simulink model "mcb_pmsm_foc_I2C_f28379d"  (R2023b)
settings: Solver=FixedStepDiscrete  StartTime=0.0  StopTime=4  RelTol=1e-3  EnableMultiTasking=on
InitFcn:
  | mcb_pmsm_foc_I2C_f28379d_data;
values from neighbouring files (symbols this model uses):
  dataType = 'single'    [mcb_pmsm_foc_I2C_f28379d_data.m]
  inverter = mcb_updateInverterParameters(pmsm,inverter,target)    [mcb_pmsm_foc_I2C_f28379d_data.m]
  PI_params = mcb_SetControllerParameters(pmsm,inverter,PU_System,T_pwm,Ts,Ts_speed)    [mcb_pmsm_foc_I2C_f28379d_data.m]
  pmsm = mcb_SetPMSMMotorParameters("SF2804")    [mcb_pmsm_foc_I2C_f28379d_data.m]
  PU_System = mcb_SetPUSystem(pmsm,inverter)    [mcb_pmsm_foc_I2C_f28379d_data.m]
  target = mcb_SetProcessorDetails('F28379D',PWM_frequency)    [mcb_pmsm_foc_I2C_f28379d_data.m]
  Ts = T_pwm    (= 5e-05)    [mcb_pmsm_foc_I2C_f28379d_data.m]
  Ts_motor = T_pwm/2    (= 2.5e-05)    [mcb_pmsm_foc_I2C_f28379d_data.m]
  Ts_sensor = 20*Ts    (= 0.001)    [mcb_pmsm_foc_I2C_f28379d_data.m]
  Ts_simulink = T_pwm/2    (= 2.5e-05)    [mcb_pmsm_foc_I2C_f28379d_data.m]
  Ts_speed = 10*Ts    (= 0.0005)    [mcb_pmsm_foc_I2C_f28379d_data.m]
undefined symbols (not defined in the file or in its folder): acceleration, DiscIntNeverNeededParam, Down, GPTRIP1SEL, GPTRIP2SEL, Speed_openLoop_PU, TZ1, TZ2, Up
libraries: c280xlib x14, simulink x12, mcbcontrolslib x9, c2802xlib x7, slpidlib x5, c2837xDlib x4, mcbpositiondecoderlib x3, canmsglib x2, svdschedulerlib x2, dspsigops x1, svdutilitieslib x1, mcbplantlib x1
(part 1 of 3)
settings Model: ExtModeTrigDuration=8  Creator=The MathWorks, Inc.  LastModifiedBy=13571
settings SolverCC: AlgebraicLoopSolver=TrustRegion  AutoInsertRateTranBlk=on  MaxZcPerStep=1
settings OptimizationCC: DefaultParameterBehavior=Inlined  DefaultUnderspecifiedDataType=single  OptimizeBlockIOStorage=off  ReuseModelBlockBuffer=off  EnhancedBackFolding=on  InitFltsAndDblsToZero=on  NoFixptDivByZeroProtection=on  EfficientFloat2IntCast=on  EfficientMapNaN2IntZero=off  MaxStackSize=1024  OptimizeBlockOrder=speed  DifferentSizesBufferReuse=on  DenormalBehavior=FlushToZero  EfficientTunableParamExpr=on
settings DebuggingCC: MultiTaskDSMMsg=none  ParameterPrecisionLossMsg=none  ParameterTunabilityLossMsg=error  UnconnectedInputMsg=warning  UnconnectedOutputMsg=warning  UnconnectedLineMsg=warning
settings HardwareCC: ProdBitPerChar=16  ProdBitPerInt=16  ProdBitPerPointer=32  ProdBitPerSizeT=32  ProdBitPerPtrDiffT=32  ProdLargestAtomicInteger=Integer  ProdLargestAtomicFloat=None  ProdWordSize=16  ProdLongLongMode=on  ProdHWDeviceType=Texas Instruments->C2000
settings ModelReferenceCC: EnableRefExpFcnMdlSchedulingChecks=on
settings SFSimCC: MATLABDynamicMemAlloc=off
settings RTWCC: Description=Embedded Coder  SystemTargetFile=ert.tlc  HardwareBoard=TI Delfino F28379D LaunchPad  TemplateMakefile=ert_default_tmf  GenerateReport=on  Toolchain=Texas Instruments Code Composer Studio (C2000)  DLArmComputeVersion=19.05
settings CodeAppCC: IgnoreCustomStorageClasses=off  StateflowObjectComments=on
settings ERTTargetCC: CodeReplacementLibrary=TI C28x  ExtModeStaticAllocSize=10000  ConvertIfToSwitch=off  SuppressUnreachableDefaultCases=off  MemSecPackage=tic2000demospkg

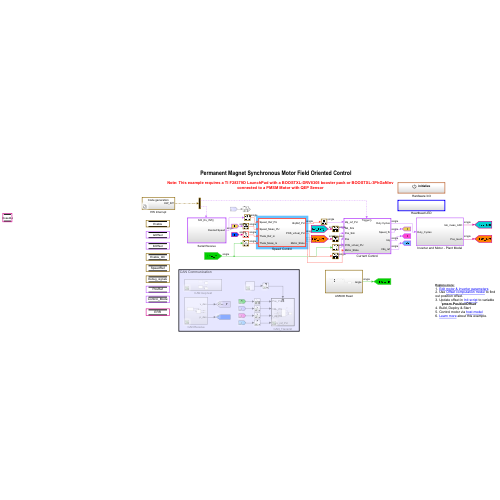
[thumbnail: Simulink's stored preview of the top-level diagram]
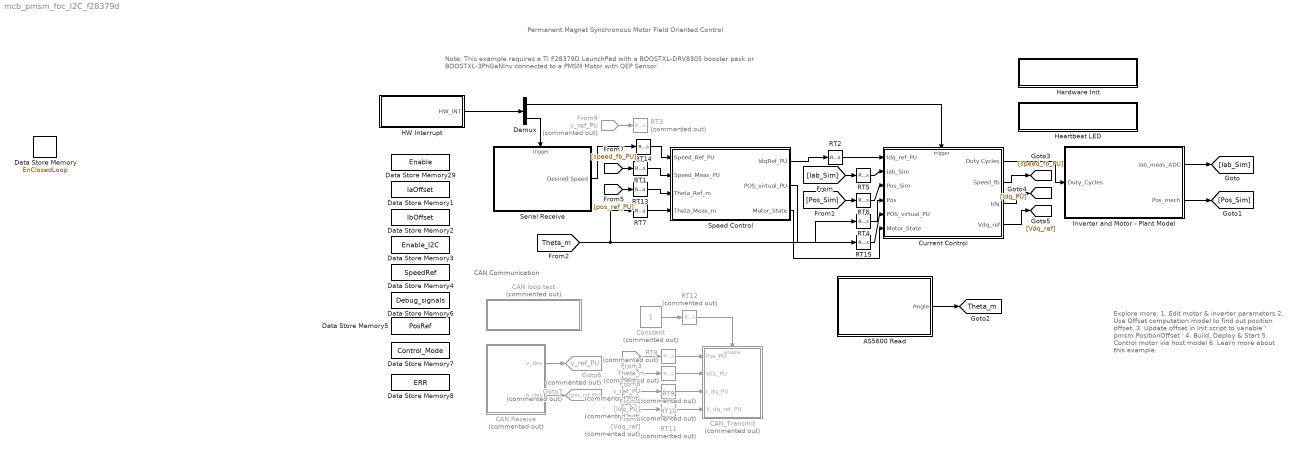
== system mcb_pmsm_foc_I2C_f28379d ==
  note: CAN Communication
  note: Note: This example requires a TI F28379D LaunchPad with a BOOSTXL-DRV8305 booster pack or BOOSTXL-3PhGaNInv
      | connected to a PMSM Motor with QEP Sensor
  note: Permanent Magnet Synchronous Motor Field Oriented Control
  note: Explore more:
      | 1. Edit motor & inverter parameters
      | 2. Use Offset computation model to find out position offset.
      | 3. Update offset in Init script to variable ' pmsm.PositionOffset '
      | 4. Build, Deploy & Start
      | 5. Control motor via host model
      | 6. Learn more about this example.
  AS5600 Read : Subsystem
  CAN Receive : Subsystem  Commented=on
  CAN loop test : Subsystem  Commented=on
  CAN_Transmit : Subsystem  Commented=on
  Constant : Constant  Commented=on  SampleTime=15e-2
  Current Control : Subsystem
      settings: RTWSystemCode=Nonreusable function
  Data Store Memory1 : DataStoreMemory  DataStoreName=IaOffset  ReadBeforeWriteMsg=warning  WriteAfterWriteMsg=warning  WriteAfterReadMsg=warning  InitialValue=inverter.CtSensAOffset  ShowAdditionalParam=off
  Data Store Memory2 : DataStoreMemory  DataStoreName=IbOffset  ReadBeforeWriteMsg=warning  WriteAfterWriteMsg=warning  WriteAfterReadMsg=warning  InitialValue=inverter.CtSensBOffset  ShowAdditionalParam=off
  Data Store Memory29 : DataStoreMemory  DataStoreName=Enable  ReadBeforeWriteMsg=warning  WriteAfterWriteMsg=warning  WriteAfterReadMsg=warning  ShowAdditionalParam=off  OutDataTypeStr=boolean
  Data Store Memory3 : DataStoreMemory  DataStoreName=Enable_I2C  ReadBeforeWriteMsg=warning  WriteAfterWriteMsg=warning  WriteAfterReadMsg=warning  ShowAdditionalParam=off  OutDataTypeStr=boolean
  Data Store Memory4 : DataStoreMemory  DataStoreName=SpeedRef  ShowAdditionalParam=off
  Data Store Memory5 : DataStoreMemory  DataStoreName=PosRef  ShowAdditionalParam=off
  Data Store Memory6 : DataStoreMemory  DataStoreName=Debug_signals  ReadBeforeWriteMsg=warning  WriteAfterWriteMsg=warning  WriteAfterReadMsg=warning  InitialValue=5  ShowAdditionalParam=off  OutDataTypeStr=uint16
  Data Store Memory7 : DataStoreMemory  DataStoreName=Control_Mode  ShowAdditionalParam=off
  Data Store Memory8 : DataStoreMemory  DataStoreName=ERR  ShowAdditionalParam=off
  Data Store Memory : DataStoreMemory  DataStoreName=EnClosedLoop  WriteAfterWriteMsg=warning  ShowAdditionalParam=off
  Demux : Demux  Outputs=2
  From3 : From  Commented=on  GotoTag=Theta_m  TagVisibility=global
  From4 : From  Commented=on  GotoTag=Idq_PU
  From6 : From  Commented=on  GotoTag=Vdq_ref
  From8 : From  Commented=on  GotoTag=v_ref_PU  TagVisibility=global
  From9 : From  Commented=on  GotoTag=v_ref_PU  TagVisibility=global
  Goto6 : Goto  Commented=on  GotoTag=v_ref_PU  TagVisibility=global
  Goto7 : Goto  Commented=on  GotoTag=pos_ref_PU
  HW Interrupt : Subsystem  Variant=on  VariantControlMode=sim codegen switching
  Hardware Init : Subsystem  TreatAsAtomicUnit=on
  Heartbeat LED : Subsystem  TreatAsAtomicUnit=on
  Inverter and Motor - Plant Model : Subsystem
  RT1 : RateTransition  Deterministic=off  OutPortSampleTime=Ts_speed
  RT{8..11} (4 alike) : RateTransition  Commented=on  Deterministic=off
  RT12 : RateTransition  Commented=on  Deterministic=off  OutPortSampleTime=1e-1
  RT13 : RateTransition  Deterministic=off  OutPortSampleTime=Ts_speed
  RT14 : RateTransition  Deterministic=off  OutPortSampleTime=Ts_speed
  RT{2,4..7,15} (6 alike) : RateTransition  Deterministic=off
  RT3 : RateTransition  Commented=on  Deterministic=off  OutPortSampleTime=Ts_speed
  Serial Receive : Subsystem  SystemSampleTime=1e-3
  Speed Control : Subsystem  TreatAsAtomicUnit=on  SystemSampleTime=Ts_speed
  tag scope: Theta_m=global
  wires:
  HW Interrupt/1(HW_INT) -> Demux/1
  RT2/1 -> Current Control/1(Idq_ref_PU)
  Demux/1 -> Current Control/Trigger
  Current Control/1(Duty Cycles) -> Inverter and Motor - Plant Model/1(Duty_Cycles)
  Demux/2 -> Serial Receive/Trigger
  Speed Control/1(IdqRef_PU) -> RT2/1
  RT1/1 -> Speed Control/2(Speed_Meas_PU)
  Inverter and Motor - Plant Model/2(Pos_mech) -> [Pos_Sim]
  Inverter and Motor - Plant Model/1(Iab_meas_ADC) -> [Iab_Sim]
  RT6/1 -> Current Control/3(Pos_Sim)
  [Iab_Sim] -> RT5/1
  RT5/1 -> Current Control/2(Iab_Sim)
  [Pos_Sim] -> RT6/1
  AS5600 Read/1(Angle) -> [Theta_m]
  RT4/1 -> Current Control/4(Pos)
  [Theta_m] -> RT4/1, RT7/1
  RT7/1 -> Speed Control/4(Theta_Meas_m)
  Constant/1 -> RT12/1
  RT8/1 -> CAN_Transmit/1(Pos_PU)
  RT11/1 -> CAN_Transmit/4(V_dq_ref_PU)
  RT10/1 -> CAN_Transmit/3(I_dq_PU)
  From6/1 -> RT11/1
  From4/1 -> RT10/1
  From8/1 -> RT9/1
  RT12/1 -> CAN_Transmit/Enable
  RT9/1 -> CAN_Transmit/2(VEL_PU)
  From3/1 -> RT8/1
  Current Control/2(Speed_fb) -> [speed_fb_PU]
  [speed_fb_PU] -> RT1/1
  Current Control/3(Idq) -> [Idq_PU]
  Current Control/4(Vdq_ref) -> [Vdq_ref]
  CAN Receive/1(v_des) -> Goto6/1
  CAN Receive/2(p_des) -> Goto7/1
  [pos_ref_PU] -> RT13/1
  RT13/1 -> Speed Control/3(Theta_Ref_m)
  From9/1 -> RT3/1
  Serial Receive/1(Desired Speed) -> RT14/1
  RT14/1 -> Speed Control/1(Speed_Ref_PU)
  Speed Control/2(POS_virtual_PU) -> RT15/1
  RT15/1 -> Current Control/5(POS_virtual_PU)
  Speed Control/3(Motor_State) -> Current Control/6(Motor_State)

== system mcb_pmsm_foc_I2C_f28379d/AS5600 Read ==
  Data Read : Subsystem
  "Data Realignment " : Subsystem
  Data Store Read : DataStoreRead  DataStoreName=Enable_I2C  IndexOptions=Index vector (dialog)  Indices=1  OutputSizes=1
  Data Store Write : DataStoreWrite  DataStoreName=Enable_I2C  IndexOptions=Index vector (dialog)  Indices=1  OutputSizes=1
  InitTrigger : Constant  Priority=10  OutDataTypeStr=boolean  SampleTime=15e-3
  Initialization : Subsystem
  Logical Operator2 : Logic  Operator=NOT  AllPortsSameDT=off  OutDataTypeStr=boolean
  RT4 : RateTransition  Deterministic=off  OutPortSampleTime=Ts_sensor
  Unit Delay : UnitDelay  SampleTime=-1  HasFrameUpgradeWarning=on
  Angle : Outport
  wires:
  Unit Delay/1 -> Data Store Write/1, Logical Operator2/1
  InitTrigger/1 -> Unit Delay/1
  Logical Operator2/1 -> Initialization/Enable
  Data Store Read/1 -> RT4/1
  Data Read/1(Out2) -> "Data Realignment "/1(In1)
  RT4/1 -> Data Read/Enable
  "Data Realignment "/1(Angle) -> Angle/1

== system mcb_pmsm_foc_I2C_f28379d/CAN Receive ==
  CAN Receive : c280xlib/CAN Receive  chipFamily=C280x  useModule=CAN_B  mailboxNo=2  messageID=257  messageType=Standard (11-bit identifier)  enableAcceptanceFiltering=off  messageIDMask=0  sampleTime=1e-3  dataType=CAN_MESSAGE_TYPE  outputAction=Output last received values  initValue=0  outputMessageID=off  outputMessageLength=off  outputMessageTimeStamp=off  postInterrupt=on  interruptLine=0
      settings: LibrarySourceBlock=c2837xDlib/CAN Receive
  Subsystem2 : Subsystem
  v_des : Outport
  p_des : Outport  Port=2
  wires:
  CAN Receive/1 -> Subsystem2/Trigger
  Subsystem2/2(p_des) -> p_des/1
  Subsystem2/1(v_des) -> v_des/1
  CAN Receive/2 -> Subsystem2/1(RawData)

== system mcb_pmsm_foc_I2C_f28379d/CAN loop test ==
  CAN Receive : c280xlib/CAN Receive  chipFamily=C280x  useModule=CAN_B  mailboxNo=2  messageID=257  messageType=Standard (11-bit identifier)  enableAcceptanceFiltering=off  messageIDMask=0  sampleTime=1e-3  dataType=CAN_MESSAGE_TYPE  outputAction=Output last received values  initValue=0  outputMessageID=off  outputMessageLength=off  outputMessageTimeStamp=off  postInterrupt=on  interruptLine=0
      settings: LibrarySourceBlock=c2837xDlib/CAN Receive
  CAN Receive1 : c280xlib/CAN Receive  Commented=on  chipFamily=C280x  useModule=CAN_B  mailboxNo=3  messageID=2  messageType=Standard (11-bit identifier)  enableAcceptanceFiltering=off  messageIDMask=0  sampleTime=2e-1  dataType=CAN_MESSAGE_TYPE  outputAction=Output last received values  initValue=0  outputMessageID=off  outputMessageLength=off  outputMessageTimeStamp=off  postInterrupt=on  interruptLine=0
      settings: LibrarySourceBlock=c2837xDlib/CAN Receive
  Subsystem1 : Subsystem  Commented=on
  Subsystem2 : Subsystem
  wires:
  CAN Receive1/2 -> Subsystem1/1(RawData)
  CAN Receive1/1 -> Subsystem1/Trigger
  CAN Receive/2 -> Subsystem2/1(RawData)
  CAN Receive/1 -> Subsystem2/Trigger

== system mcb_pmsm_foc_I2C_f28379d/CAN_Transmit ==
  Pos_PU : Inport
  VEL_PU : Inport  Port=2
  I_dq_PU : Inport  Port=3
  V_dq_ref_PU : Inport  Port=4
  Enable : EnablePort
  CAN_Tx : Subsystem
  DataLog : Subsystem
  Demux1 : Demux  Outputs=2
  Demux2 : Demux  Outputs=2
  Gain : Gain  Gain=PU_System.I_base
  Gain1 : Gain  Gain=PU_System.I_base
  Gain2 : Gain  Gain=1/PU_System.V_base
  Gain3 : Gain  Gain=1/PU_System.V_base
  wires:
  Gain1/1 -> DataLog/4(Iq)
  DataLog/3(T_CAN) -> CAN_Tx/3(T_CAN)
  Demux1/2 -> Gain1/1
  Pos_PU/1 -> DataLog/1(Pos_PU)
  VEL_PU/1 -> DataLog/2(VEL_PU)
  Demux2/2 -> Gain3/1
  DataLog/1(POS_CAN) -> CAN_Tx/1(POS_CAN)
  Gain2/1 -> DataLog/5(Vd)
  I_dq_PU/1 -> Demux1/1
  DataLog/2(VEL_CAN) -> CAN_Tx/2(VEL_CAN)
  Demux1/1 -> Gain/1
  V_dq_ref_PU/1 -> Demux2/1
  Gain3/1 -> DataLog/6(Vq)
  Gain/1 -> DataLog/3(Id)
  Demux2/1 -> Gain2/1

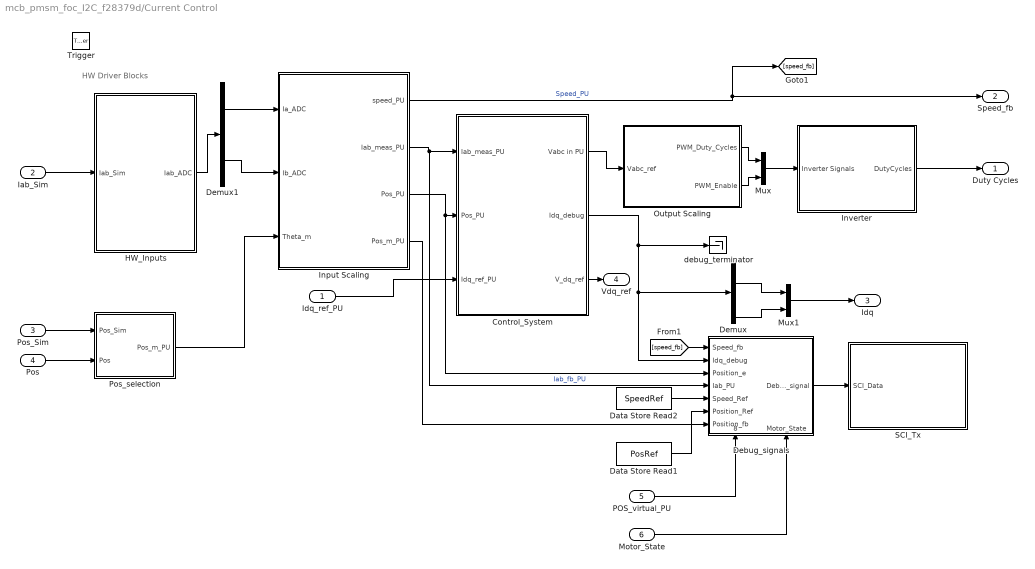
== system mcb_pmsm_foc_I2C_f28379d/Current Control ==
  note: HW Driver Blocks
  Idq_ref_PU : Inport
  Iab_Sim : Inport  Port=2
  Pos_Sim : Inport  Port=3
  Pos : Inport  Port=4
  POS_virtual_PU : Inport  Port=5
  Motor_State : Inport  Port=6
  Trigger : TriggerPort  TriggerType=function-call  VariantControl=Variant  PortDimensions=1
  Control_System : Subsystem
  Data Store Read1 : DataStoreRead  DataStoreName=PosRef  IndexOptions=Index vector (dialog)  Indices=1  OutputSizes=1
  Data Store Read2 : DataStoreRead  DataStoreName=SpeedRef  IndexOptions=Index vector (dialog)  Indices=1  OutputSizes=1
  Debug_signals : Subsystem
      settings: PortSchema="{\"entries\":[{\"content\":{\"sides\":[{\"content\":{\"connectorIds\":[\"In1\",\"In2\",\"In3\",\"In4\",\"In5\",\"In6\",\"In7\"]},\"type\":\"ConnectorPlacement.EquallySpacedRectSide\",\"uuid\":\"c3c156a1-44f3-4462-a7bb-0816c19c2a97\"},{\"content\":{\"connectorIds\":[\"Out1\"],\"side\":\"RIGHT\"},\"type\":\"ConnectorPlacement.EquallySpacedRectSide\",\"uuid\":\"dea011ce-0ad1-4d3a-bd12-401efdcd125e\"},{\"content\":{\"side\":\"TOP\"},\"type\":\"ConnectorPlacement.EquallySpacedRectSide\",\"uuid\":\"b5c47e72-5d5f-45aa-96da-a691da1944bd\"},{\"content\":{\"connectorIds\":[\"In8\",\"In9\"],\"side\":\"BOTTOM\"},\"type\":\"ConnectorPlacement.EquallySpacedRectSide\",\"uuid\":\"0e9b7920-397e-4ec1-b840-59fd6ccb72da\"}]},\"type\":\"ConnectorPlacement.EquallySpacedConnector\",\"uuid\":\"99cda5f3-8c4e-43f6-994a-d197feadfb64\"}],\"packageUris\":[\"http://schema.mathworks.com/mf0/Connector/R2020b\"],\"version\":\"1.0\"}"
  Demux : Demux
  Demux1 : Demux  Outputs=2
  HW_Inputs : Subsystem  Variant=on  VariantControlMode=sim codegen switching
  Input Scaling : Subsystem
  Inverter : Subsystem  Variant=on  VariantControlMode=sim codegen switching
  Mux : Mux  Inputs=2
  Mux1 : Mux  Inputs=2
  Output Scaling : Subsystem
  Pos_selection : Subsystem  Variant=on  VariantControlMode=sim codegen switching
  SCI_Tx : Subsystem  Variant=on  VariantControlMode=sim codegen switching
  debug_terminator : Terminator
  Duty Cycles : Outport  InitialOutput=0  VectorParamsAs1DForOutWhenUnconnected=off
  Speed_fb : Outport  Port=2  InitialOutput=0  VectorParamsAs1DForOutWhenUnconnected=off
  Idq : Outport  Port=3  InitialOutput=0  VectorParamsAs1DForOutWhenUnconnected=off
  Vdq_ref : Outport  Port=4  InitialOutput=0  VectorParamsAs1DForOutWhenUnconnected=off
  wires:
  Input Scaling/3(Pos_PU) -> Debug_signals/3(Position_e), Control_System/2(Pos_PU)
  Idq_ref_PU/1 -> Control_System/3(Idq_ref_PU)
  Input Scaling/1(speed_PU) -> [speed_fb], Speed_fb/1  "Speed_PU"
  Input Scaling/2(Iab_meas_PU) -> Debug_signals/4(Iab_PU), Control_System/1(Iab_meas_PU)  "Iab_fb_PU"
  Demux1/1 -> Input Scaling/1(Ia_ADC)
  Demux1/2 -> Input Scaling/2(Ib_ADC)
  Output Scaling/1(PWM_Duty_Cycles) -> Mux/1
  Debug_signals/1(Debug_signal) -> SCI_Tx/1(SCI_Data)
  Mux/1 -> Inverter/1(Inverter Signals)
  Output Scaling/2(PWM_Enable) -> Mux/2
  Inverter/1(DutyCycles) -> Duty Cycles/1
  HW_Inputs/1(Iab_ADC) -> Demux1/1
  Pos_Sim/1 -> Pos_selection/1(Pos_Sim)
  Control_System/1(Vabc in PU) -> Output Scaling/1(Vabc_ref)
  Iab_Sim/1 -> HW_Inputs/1(Iab_Sim)
  Data Store Read2/1 -> Debug_signals/5(Speed_Ref)
  [speed_fb] -> Debug_signals/1(Speed_fb)
  Data Store Read1/1 -> Debug_signals/6(Position_Ref)
  Input Scaling/4(Pos_m_PU) -> Debug_signals/7(Position_fb)
  Pos/1 -> Pos_selection/2(Pos)
  Pos_selection/1(Pos_m_PU) -> Input Scaling/3(Theta_m)
  Control_System/2(Idq_debug) -> Debug_signals/2(Idq_debug), Demux/1, debug_terminator/1
  Demux/2 -> Mux1/1
  Demux/4 -> Mux1/2
  Mux1/1 -> Idq/1
  Control_System/3(V_dq_ref) -> Vdq_ref/1
  POS_virtual_PU/1 -> Debug_signals/8(POS_virtual_PU)
  Motor_State/1 -> Debug_signals/9(Motor_State)

== system mcb_pmsm_foc_I2C_f28379d/HW Interrupt ==
  Code generation : Subsystem  VariantControl=(codegen)
  Simulation : Subsystem  VariantControl=(sim)
  HW_INT : Outport  OutputFunctionCall=on

== system mcb_pmsm_foc_I2C_f28379d/Hardware Init ==
  6PWM_Mode : Constant  Priority=1000  Value=0x3A16  OutDataTypeStr=uint16  SampleTime=-1
  ADC_Gain_Setting : Constant  Priority=1000  Value=inverter.SPI_Gain_Setting  OutDataTypeStr=uint16  SampleTime=-1
  Event Listener : EventListener  DisableCoverage=on  EventName=reset
  Mux : Mux  Inputs=2
  Variant Subsystem : Subsystem  Variant=on  VariantControlMode=sim codegen switching
  wires:
  6PWM_Mode/1 -> Mux/1
  ADC_Gain_Setting/1 -> Mux/2
  Mux/1 -> Variant Subsystem/1(In1)

== system mcb_pmsm_foc_I2C_f28379d/Heartbeat LED ==
  note: Heartbeat LED 1HZ
  Heartbeat LED : Subsystem  Variant=on  VariantControlMode=sim codegen switching
  RED_LED : Constant  OutDataTypeStr=uint16  SampleTime=0.5
  wires:
  RED_LED/1 -> Heartbeat LED/1(In1)

== system mcb_pmsm_foc_I2C_f28379d/Inverter and Motor - Plant Model ==
  Duty_Cycles : Inport
  Codegeneration : Subsystem
  Simulation : Subsystem
  Variant Sink : VariantSink  VariantControlMode=sim codegen switching
  Variant Source1 : VariantSource  VariantControlMode=sim codegen switching
  Variant Source2 : VariantSource  VariantControlMode=sim codegen switching
  Iab_meas_ADC : Outport  VectorParamsAs1DForOutWhenUnconnected=off
  Pos_mech : Outport  Port=2  VectorParamsAs1DForOutWhenUnconnected=off
  wires:
  Duty_Cycles/1 -> Variant Sink/1
  Variant Sink/2 -> Simulation/1(Duty_Cycles)
  Variant Sink/1 -> Codegeneration/1(Duty_Cycles)
  Codegeneration/2(Pos_fb_Sim) -> Variant Source2/1
  Codegeneration/1(Iab_fb_Sim) -> Variant Source1/1
  Variant Source1/1 -> Iab_meas_ADC/1
  Simulation/2(Pos_fb_Sim) -> Variant Source2/2
  Simulation/1(Iab_fb_Sim) -> Variant Source1/2
  Variant Source2/1 -> Pos_mech/1

== system mcb_pmsm_foc_I2C_f28379d/Serial Receive ==
  SCI_Rx_INT : TriggerPort  TriggerType=function-call  VariantControl=Variant
  Data Store Write : DataStoreWrite  DataStoreName=Enable  IndexOptions=Index vector (dialog)  Indices=1  OutputSizes=1
  Data Store Write1 : DataStoreWrite  DataStoreName=SpeedRef  IndexOptions=Index vector (dialog)  Indices=1  OutputSizes=1
  Data Store Write2 : DataStoreWrite  DataStoreName=Debug_signals  IndexOptions=Index vector (dialog)  Indices=1  OutputSizes=1
  Data Store Write3 : DataStoreWrite  DataStoreName=Control_Mode  IndexOptions=Index vector (dialog)  Indices=1  OutputSizes=1
  Data_Conditioning_Rx : Subsystem  Variant=on
  SCI_Rx : Subsystem  Variant=on  VariantControlMode=sim codegen switching
  unParse : Subsystem
  Desired Speed : Outport  VectorParamsAs1DForOutWhenUnconnected=off
  wires:
  unParse/2(Debug_signals) -> Data Store Write2/1
  Data_Conditioning_Rx/2(Out2) -> unParse/1(Data)
  SCI_Rx/1(Data) -> Data_Conditioning_Rx/1(In1)
  unParse/1(Enable_PWM) -> Data Store Write/1
  unParse/3(Control_Mode) -> Data Store Write3/1
  Data_Conditioning_Rx/1(Desired Speed) -> Data Store Write1/1, Desired Speed/1

== system mcb_pmsm_foc_I2C_f28379d/Speed Control ==
  Speed_Ref_PU : Inport
  Speed_Meas_PU : Inport  Port=2
  Theta_Ref_m : Inport  Port=3
  Theta_Meas_m : Inport  Port=4
  Id_ref : Constant  Value=0  OutDataTypeStr=dataType  SampleTime=Ts_speed
  Mux1 : Mux  Inputs=2
  PI_Controller_Speed : Subsystem
  PI_Controller_Speed1 : Subsystem  Commented=on
  POS_Loop : Subsystem  Commented=on
  SlewRate : Subsystem  Commented=on
  Speed_Ref_Selector : Subsystem
  IdqRef_PU : Outport  VectorParamsAs1DForOutWhenUnconnected=off
  POS_virtual_PU : Outport  Port=2  VectorParamsAs1DForOutWhenUnconnected=off
  Motor_State : Outport  Port=3  VectorParamsAs1DForOutWhenUnconnected=off
  wires:
  Speed_Meas_PU/1 -> PI_Controller_Speed/2(N_fb), Speed_Ref_Selector/2(Speed_Ref_Open)  "Speed_fb"
  Id_ref/1 -> Mux1/1
  Mux1/1 -> IdqRef_PU/1
  Theta_Meas_m/1 -> POS_Loop/2(Theta_fb)
  Theta_Ref_m/1 -> POS_Loop/1(Theta_ref)
  Speed_Ref_PU/1 -> Speed_Ref_Selector/1(Speed_Ref_In), POS_Loop/3(Speed_Ref_PU)
  Speed_Ref_Selector/1(Speed_Ref_PU) -> PI_Controller_Speed/1(N_ref)  "Speed_Ref"
  PI_Controller_Speed/1(Iq_ref) -> Mux1/2

== system mcb_pmsm_foc_I2C_f28379d/AS5600 Read/Data Read ==
  Enable : EnablePort
  Data Read Adress : Constant  Priority=10  Value=hex2dec('0E')  OutDataTypeStr=uint8  SampleTime=-1
  I2C Receive : c280xlib/I2C Receive  Priority=10  selectModule=I2C_A  addrFormat=7-Bit addressing  saSource=Input port  SAR=54  bitCount=8  dataLength=2  initValue=0  NACK=off  STP=on  STR=on  sampleTime=-1  dataType=uint8
  I2C Transmit : c280xlib/I2C Transmit  Priority=20  selectModule=I2C_A  addrFormat=7-Bit addressing  saSource=Input port  SAR=0x36  bitCount=8  STP=off  RM=off  STR=on
  Register Address : Constant  Value=hex2dec('0x36')  OutDataTypeStr=uint8  SampleTime=-1
  Terminator : Terminator
  Terminator1 : Terminator
  Out2 : Outport  VectorParamsAs1DForOutWhenUnconnected=off
  wires:
  I2C Transmit/1 -> Terminator/1
  I2C Receive/1 -> Out2/1
  I2C Receive/2 -> Terminator1/1
  Data Read Adress/1 -> I2C Transmit/2
  Register Address/1 -> I2C Transmit/1, I2C Receive/1

== system mcb_pmsm_foc_I2C_f28379d/AS5600 Read/Data Realignment  ==
  In1 : Inport
  Cast To Single : DataTypeConversion  OutDataTypeStr=single  SaturateOnIntegerOverflow=off  RndMeth=Floor
  Cast To Single1 : DataTypeConversion  OutDataTypeStr=single  SaturateOnIntegerOverflow=off  RndMeth=Floor
  Constant : Constant
  Gain : Gain  Gain=1/4096
  MATLAB Function : MATLAB Function  TreatAsAtomicUnit=on
  Reshape : Reshape  OutputDimensionality=Customize  OutputDimensions=[2,1]
  Sum : Sum  Inputs=|-+
  Angle : Outport  VectorParamsAs1DForOutWhenUnconnected=off
  wires:
  In1/1 -> Reshape/1
  Reshape/1 -> MATLAB Function/1(data)
  MATLAB Function/1(raw_angle) -> Cast To Single1/1
  Cast To Single/1 -> Angle/1
  Cast To Single1/1 -> Gain/1
  Constant/1 -> Sum/2
  Gain/1 -> Cast To Single/1

== system mcb_pmsm_foc_I2C_f28379d/AS5600 Read/Initialization ==
  Enable : EnablePort
  Address - Data read : Subsystem  TreatAsAtomicUnit=on
  Delay 1ms : Subsystem  TreatAsAtomicUnit=on
  Function-Call Generator : simulink/Ports & Subsystems/Function-Call Generator  sample_time=-1  numberOfIterations=1  DisallowWideOutput=off
  Function-Call Split1 : FunctionCallSplit  NumOutputPorts=2
  wires:
  Function-Call Generator/1 -> Function-Call Split1/1
  Function-Call Split1/1 -> Address - Data read/Trigger
  Function-Call Split1/2 -> Delay 1ms/Trigger

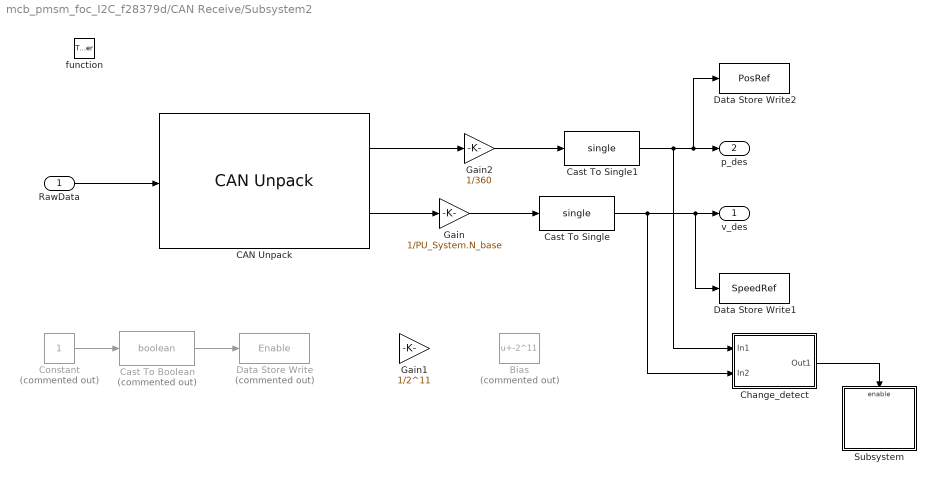
== system mcb_pmsm_foc_I2C_f28379d/CAN Receive/Subsystem2 ==
  RawData : Inport
  function : TriggerPort  TriggerType=function-call  VariantControl=(inherit)
  Bias : Bias  Commented=on  Bias=-2^11  SaturateOnIntegerOverflow=off
  CAN Unpack : canmsglib/CAN Unpack  CANdbFile=D:\project\internship\mcb\FOCI2CExample\motor_can.dbc  MsgList=POS_VEL_Control  MsgName=POS_VEL_Control  MsgIDType=Standard (11-bit identifier)  MsgIdentifier=257  MsgLength=8  SignalInfo={'p_des','24','32','BE','single','Standard','0','1','0','-3.4e+38','3.4e+38';'v_des','32','32','LE','single','Standard','0','1','0','-3.4e+38','3.4e+38'}  IDPort=off  TimestampPort=off  ErrorPort=off  RemotePort=off  LengthPort=off  StatusPort=off  ApplyMinMax=off
      settings: LibrarySourceBlock=c2000lib/Target Communication/CAN Unpack  DataFormat=CANdb specified signals
  Cast To Boolean : DataTypeConversion  Commented=on  OutDataTypeStr=boolean  SaturateOnIntegerOverflow=off  RndMeth=Floor
  Cast To Single : DataTypeConversion  OutDataTypeStr=single  SaturateOnIntegerOverflow=off  RndMeth=Floor
  Cast To Single1 : DataTypeConversion  OutDataTypeStr=single  SaturateOnIntegerOverflow=off  RndMeth=Floor
  Change_detect : Subsystem
  Constant : Constant  Commented=on
  Data Store Write : DataStoreWrite  Commented=on  DataStoreName=Enable  IndexOptions=Index vector (dialog)  Indices=1  OutputSizes=1
  Data Store Write1 : DataStoreWrite  DataStoreName=SpeedRef  IndexOptions=Index vector (dialog)  Indices=1  OutputSizes=1
  Data Store Write2 : DataStoreWrite  DataStoreName=PosRef  IndexOptions=Index vector (dialog)  Indices=1  OutputSizes=1
  Gain : Gain  Gain=1/PU_System.N_base
  Gain1 : Gain  Gain=1/2^11
  Gain2 : Gain  Gain=1/360
  Subsystem : Subsystem
  v_des : Outport
  p_des : Outport  Port=2
  wires:
  RawData/1 -> CAN Unpack/1
  Constant/1 -> Cast To Boolean/1
  Cast To Boolean/1 -> Data Store Write/1
  CAN Unpack/2 -> Gain/1
  Gain/1 -> Cast To Single/1
  Cast To Single/1 -> Change_detect/2(In2), Data Store Write1/1, v_des/1
  Change_detect/1(Out1) -> Subsystem/Enable
  CAN Unpack/1 -> Gain2/1
  Gain2/1 -> Cast To Single1/1
  Cast To Single1/1 -> Change_detect/1(In1), Data Store Write2/1, p_des/1

== system mcb_pmsm_foc_I2C_f28379d/CAN loop test/Subsystem1 ==
  RawData : Inport
  function : TriggerPort  TriggerType=function-call  VariantControl=(inherit)
  CAN Transmit1 : c280xlib/CAN Transmit  chipFamily=C280x  useModule=CAN_B  mailboxNo=1  messageID=2  messageType=Standard (11-bit identifier)  enableBlockingMode=off  postInterrupt=on  interruptLine=0
      settings: LibrarySourceBlock=c280015xlib/CAN Transmit
  wires:
  RawData/1 -> CAN Transmit1/1

== system mcb_pmsm_foc_I2C_f28379d/CAN loop test/Subsystem2 ==
  RawData : Inport
  function : TriggerPort  TriggerType=function-call  VariantControl=(inherit)
  CAN Transmit1 : c280xlib/CAN Transmit  chipFamily=C280x  useModule=CAN_B  mailboxNo=1  messageID=2  messageType=Standard (11-bit identifier)  enableBlockingMode=off  postInterrupt=on  interruptLine=0
      settings: LibrarySourceBlock=c280015xlib/CAN Transmit
  wires:
  RawData/1 -> CAN Transmit1/1

== system mcb_pmsm_foc_I2C_f28379d/CAN_Transmit/CAN_Tx ==
  POS_CAN : Inport
  VEL_CAN : Inport  Port=2
  T_CAN : Inport  Port=3
  CAN Pack : canmsglib/CAN Pack  CANdbFile=D:\project\internship\mcb\FOCI2CExample\motor_can.dbc  MsgList=PMSMFeedback  MsgName=PMSMFeedback  MsgIDType=Standard (11-bit identifier)  MsgIdentifier=17  MsgLength=8  Remote=off  ApplyMinMax=off  BusOutput=off  SignalInfo={'ERR','0','4','BE','unsigned','Standard','0','1','0','0','15';'ID','4','4','BE','unsigned','Standard','0','1','0','0','15';'POS','16','16','BE','unsigned','Standard','0','1','0','0','65535';'T','40','12','BE','unsigned','Standard','0','1','0','0','4095';'T_MOS','48','8','BE','unsigned','Standard','0','1','0','0','255';'T_Rotor','56','8','BE','unsigned','Standard','0','1','0','0','255';'VEL','36','12','BE','unsigned','Standard','0','1','0','0','4095'}
      settings: LibrarySourceBlock=c2000lib/Target Communication/CAN Pack  DataFormat=CANdb specified signals
  CAN Transmit1 : c280xlib/CAN Transmit  chipFamily=C280x  useModule=CAN_B  mailboxNo=1  messageID=17  messageType=Standard (11-bit identifier)  enableBlockingMode=off  postInterrupt=on  interruptLine=1
      settings: LibrarySourceBlock=c280015xlib/CAN Transmit
  Data Store Read1 : DataStoreRead  DataStoreName=ERR  IndexOptions=Index vector (dialog)  Indices=1  OutputSizes=1
  Data Type Conversion{,1,5..6} (4 alike) : DataTypeConversion  OutDataTypeStr=uint16  SaturateOnIntegerOverflow=off  RndMeth=Floor
  ID : Constant  Value=0x1
  T_MOS : Constant  Value=0
  T_Rotor : Constant  Value=0
  wires:
  Data Store Read1/1 -> Data Type Conversion1/1
  ID/1 -> Data Type Conversion/1
  T_MOS/1 -> Data Type Conversion5/1
  T_Rotor/1 -> Data Type Conversion6/1
  POS_CAN/1 -> CAN Pack/3
  CAN Pack/1 -> CAN Transmit1/1
  Data Type Conversion/1 -> CAN Pack/2
  Data Type Conversion1/1 -> CAN Pack/1
  T_CAN/1 -> CAN Pack/4
  Data Type Conversion5/1 -> CAN Pack/5
  Data Type Conversion6/1 -> CAN Pack/6
  VEL_CAN/1 -> CAN Pack/7

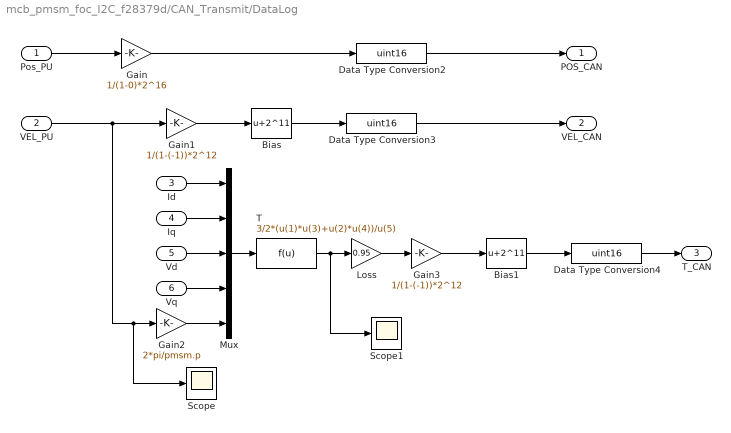
== system mcb_pmsm_foc_I2C_f28379d/CAN_Transmit/DataLog ==
  Pos_PU : Inport
  VEL_PU : Inport  Port=2
  Id : Inport  Port=3
  Iq : Inport  Port=4
  Vd : Inport  Port=5
  Vq : Inport  Port=6
  Bias : Bias  Bias=2^11  SaturateOnIntegerOverflow=off
  Bias1 : Bias  Bias=2^11  SaturateOnIntegerOverflow=off
  Data Type Conversion2 : DataTypeConversion  OutDataTypeStr=uint16  SaturateOnIntegerOverflow=off  RndMeth=Floor
  Data Type Conversion3 : DataTypeConversion  OutDataTypeStr=uint16  SaturateOnIntegerOverflow=off  RndMeth=Floor
  Data Type Conversion4 : DataTypeConversion  OutDataTypeStr=uint16  SaturateOnIntegerOverflow=off  RndMeth=Floor
  Gain : Gain  Gain=1/(1-0)*2^16
  Gain1 : Gain  Gain=1/(1-(-1))*2^12
  Gain2 : Gain  Gain=2*pi/pmsm.p
  Gain3 : Gain  Gain=1/(1-(-1))*2^12
  Loss : Gain  Gain=0.95
  Mux : Mux  Inputs=5
  Scope : Scope
  Scope1 : Scope
  T : Fcn  Expr=3/2*(u(1)*u(3)+u(2)*u(4))/u(5)
  POS_CAN : Outport
  VEL_CAN : Outport  Port=2
  T_CAN : Outport  Port=3
  wires:
  Pos_PU/1 -> Gain/1
  VEL_PU/1 -> Gain1/1, Scope/1, Gain2/1
  Mux/1 -> T/1
  Id/1 -> Mux/1
  Iq/1 -> Mux/2
  Vd/1 -> Mux/3
  Vq/1 -> Mux/4
  Gain2/1 -> Mux/5
  Gain3/1 -> Bias1/1
  Gain/1 -> Data Type Conversion2/1
  Data Type Conversion2/1 -> POS_CAN/1
  Data Type Conversion4/1 -> T_CAN/1
  T/1 -> Scope1/1, Loss/1
  Loss/1 -> Gain3/1
  Bias1/1 -> Data Type Conversion4/1
  Data Type Conversion3/1 -> VEL_CAN/1
  Gain1/1 -> Bias/1
  Bias/1 -> Data Type Conversion3/1

== system mcb_pmsm_foc_I2C_f28379d/Current Control/Control_System ==
  Iab_meas_PU : Inport
  Pos_PU : Inport  Port=2
  Idq_ref_PU : Inport  Port=3
  Clarke Transform : mcbcontrolslib/Clarke Transform  VariantControl=Variant2  PhaseInput=Two inputs  EnPowerInv=off
  Current_Controllers : Subsystem
  Demux : Demux  Outputs=2
  Inverse Park Transform : mcbcontrolslib/Inverse Park Transform  PhaseInput=Two inputs  AxisAlignment=D-axis  ThetaInput=Electrical position  AngleInput=Per-unit  N_points=1024
  Mux : Mux  Inputs=2
  Mux1 : Mux  Inputs=3
  Park Transform : mcbcontrolslib/Park Transform  PhaseInput=Two inputs  AxisAlignment=D-axis  ThetaInput=Electrical position  AngleInput=Per-unit  N_points=1024
  Space Vector Generator : mcbcontrolslib/PWM Reference Generator  inSignal=Valphabeta  modType=SVM: space vector modulation
  Vabc in PU : Outport  VectorParamsAs1DForOutWhenUnconnected=off
  Idq_debug : Outport  Port=2  VectorParamsAs1DForOutWhenUnconnected=off
  V_dq_ref : Outport  Port=3
  wires:
  Clarke Transform/2 -> Park Transform/2
  Clarke Transform/1 -> Park Transform/1
  Current_Controllers/3(Idq) -> Idq_debug/1
  Space Vector Generator/2 -> Mux1/2
  Idq_ref_PU/1 -> Current_Controllers/3(Ida_ref_PU)
  Mux1/1 -> Vabc in PU/1
  Inverse Park Transform/2 -> Space Vector Generator/2
  Inverse Park Transform/1 -> Space Vector Generator/1
  Demux/1 -> Clarke Transform/1
  Park Transform/1 -> Current_Controllers/1(Id)
  Pos_PU/1 -> Inverse Park Transform/3, Park Transform/3
  Space Vector Generator/1 -> Mux1/1
  Space Vector Generator/3 -> Mux1/3
  Park Transform/2 -> Current_Controllers/2(Iq)
  Demux/2 -> Clarke Transform/2
  Iab_meas_PU/1 -> Demux/1
  Mux/1 -> V_dq_ref/1
  Current_Controllers/1(Vd_ref) -> Mux/1, Inverse Park Transform/1
  Current_Controllers/2(Vq_ref) -> Mux/2, Inverse Park Transform/2

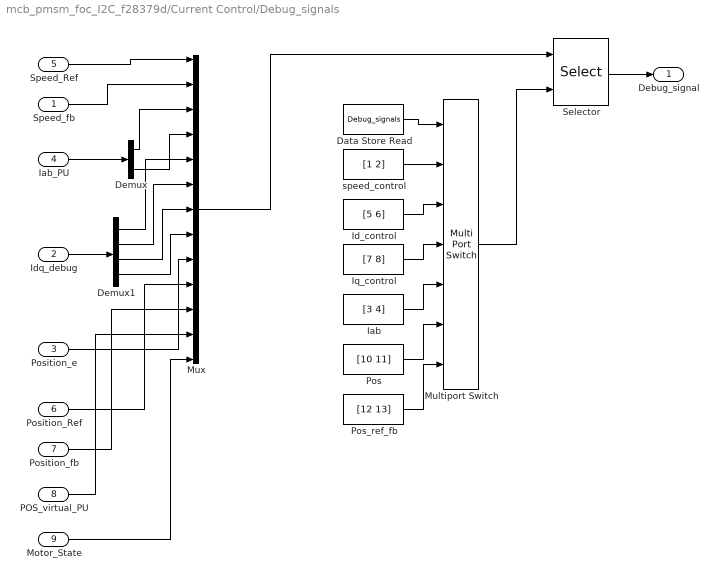
== system mcb_pmsm_foc_I2C_f28379d/Current Control/Debug_signals ==
  Speed_fb : Inport
  Idq_debug : Inport  Port=2
  Position_e : Inport  Port=3
  Iab_PU : Inport  Port=4
  Speed_Ref : Inport  Port=5
  Position_Ref : Inport  Port=6
  Position_fb : Inport  Port=7
  POS_virtual_PU : Inport  Port=8
  Motor_State : Inport  Port=9
  Data Store Read : DataStoreRead  DataStoreName=Debug_signals  IndexOptions=Index vector (dialog)  Indices=1  OutputSizes=1
  Demux : Demux  Outputs=2
  Demux1 : Demux
  Iab : Constant  Value=[3 4]  OutDataTypeStr=uint16  SampleTime=-1
  Id_control : Constant  Value=[5 6]  OutDataTypeStr=uint16  SampleTime=-1
  Iq_control : Constant  Value=[7 8]  OutDataTypeStr=uint16  SampleTime=-1
  Multiport Switch : MultiPortSwitch  Inputs=6  DiagnosticForDefault=Warning  OutDataTypeStr=uint16  RndMeth=Simplest  SaturateOnIntegerOverflow=off  InputSameDT=off
  Mux : Mux  Inputs=13
  Pos : Constant  Value=[10 11]  OutDataTypeStr=uint16  SampleTime=-1
  Pos_ref_fb : Constant  Value=[12 13]  OutDataTypeStr=uint16  SampleTime=-1
  Selector : Selector  InputPortWidth=13  IndexOptions=Index vector (port)  Indices=[1 3]  OutputSizes=1
  speed_control : Constant  Value=[1 2]  OutDataTypeStr=uint16  SampleTime=-1
  Debug_signal : Outport
  wires:
  speed_control/1 -> Multiport Switch/2
  Id_control/1 -> Multiport Switch/3
  Iq_control/1 -> Multiport Switch/4
  Iab/1 -> Multiport Switch/5
  Pos/1 -> Multiport Switch/6
  Multiport Switch/1 -> Selector/2
  Data Store Read/1 -> Multiport Switch/1
  Selector/1 -> Debug_signal/1
  Iab_PU/1 -> Demux/1
  Demux/1 -> Mux/3
  Demux/2 -> Mux/4
  Demux1/1 -> Mux/5
  Demux1/2 -> Mux/6
  Demux1/3 -> Mux/7
  Demux1/4 -> Mux/8
  Idq_debug/1 -> Demux1/1
  Mux/1 -> Selector/1
  Position_e/1 -> Mux/9
  Speed_Ref/1 -> Mux/1
  Speed_fb/1 -> Mux/2
  Pos_ref_fb/1 -> Multiport Switch/7
  Position_Ref/1 -> Mux/10
  Position_fb/1 -> Mux/11
  POS_virtual_PU/1 -> Mux/12
  Motor_State/1 -> Mux/13

== system mcb_pmsm_foc_I2C_f28379d/Current Control/HW_Inputs ==
  Iab_Sim : Inport
  Sensor Driver Blocks (codegen) : Subsystem  VariantControl=(codegen)
  Sensor Driver Blocks (sim) : Subsystem  VariantControl=(sim)
  Iab_ADC : Outport

== system mcb_pmsm_foc_I2C_f28379d/Current Control/Input Scaling ==
  note: Current Measurements
  note: Position & Speed Measurements
  note: AS5600(I2C communication)
  Ia_ADC : Inport
  Ib_ADC : Inport  Port=2
  Theta_m : Inport  Port=3
  " Calculate Position and Speed" : Subsystem
  Calculate Phase Currents : Subsystem
  speed_PU : Outport
  Iab_meas_PU : Outport  Port=2
  Pos_PU : Outport  Port=3
  Pos_m_PU : Outport  Port=4
  wires:
  " Calculate Position and Speed"/3(speed) -> speed_PU/1
  Calculate Phase Currents/1(Iab_meas_PU) -> Iab_meas_PU/1  "Iab_fb_PU"
  " Calculate Position and Speed"/1(Theta_e) -> Pos_PU/1
  Ia_ADC/1 -> Calculate Phase Currents/1(Ia_ADC)
  Ib_ADC/1 -> Calculate Phase Currents/2(Ib_ADC)
  Theta_m/1 -> " Calculate Position and Speed"/1(Theta_m)
  " Calculate Position and Speed"/2(Pos_m_PU) -> Pos_m_PU/1

== system mcb_pmsm_foc_I2C_f28379d/Current Control/Inverter ==
  Inverter Signals : Inport
  Code Generation : Subsystem  VariantControl=(codegen)
  Simulation : Subsystem  VariantControl=(sim)
  DutyCycles : Outport  VectorParamsAs1DForOutWhenUnconnected=off

== system mcb_pmsm_foc_I2C_f28379d/Current Control/Output Scaling ==
  Vabc_ref : Inport
  Constant : Constant  Value=0.5  OutDataTypeStr=dataType  SampleTime=-1
  Data Type Conversion : DataTypeConversion  OutDataTypeStr=dataType  SaturateOnIntegerOverflow=off  RndMeth=Floor
  Enable : DataStoreRead  DataStoreName=Enable  IndexOptions=Index vector (dialog)  Indices=1  OutputSizes=1
  One_by_Two : Gain  Gain=0.5  RndMeth=Simplest  OutDataTypeStr=Inherit: Same as input
  Sum : Sum  Inputs=|++
  PWM_Duty_Cycles : Outport
  PWM_Enable : Outport  Port=2
  wires:
  Constant/1 -> Sum/2
  Vabc_ref/1 -> One_by_Two/1
  Sum/1 -> PWM_Duty_Cycles/1  "PWM_Duty_Cycles"
  Enable/1 -> Data Type Conversion/1  "PWM_En"
  One_by_Two/1 -> Sum/1
  Data Type Conversion/1 -> PWM_Enable/1

== system mcb_pmsm_foc_I2C_f28379d/Current Control/Pos_selection ==
  Pos_Sim : Inport
  Pos : Inport  Port=2
  Sensor Driver Blocks (codegen) : Subsystem  VariantControl=(codegen)
  Sensor Driver Blocks (sim) : Subsystem  VariantControl=(sim)
  Pos_m_PU : Outport

== system mcb_pmsm_foc_I2C_f28379d/Current Control/SCI_Tx ==
  SCI_Data : Inport
  Code Generation : Subsystem  VariantControl=(codegen)
  Simulation : Subsystem  VariantControl=(sim)

== system mcb_pmsm_foc_I2C_f28379d/HW Interrupt/Code generation ==
  HWI_ADCB1_INT : svdschedulerlib/Hardware Interrupt v2  ISRGroup=ADC - Analog to Digital Converter  ISRName=ADCA1_INT  ISRNumber=32  NumEventsToServe=1  EventsList={'on','EOC event','1';'off','Overflow event','2';'off','Custom event','3'}  SelectedEvents={'event1'}  TaskPriority=30  DisablePreemption=off  ClearInterruptFlagsAtEndOfEvent=on  InterruptDefinitionFile=$(TARGET_ROOT)/registry/interrupts/F2837xS_interrupts.xml  HardwareBoard=F2837x  EnableSimPort=off
      settings: LibrarySourceBlock=c2000lib/Scheduling/Hardware Interrupt
  HWI_SCIA_RX_INT : svdschedulerlib/Hardware Interrupt v2  ISRGroup=ADC - Analog to Digital Converter  ISRName=ADCA1_INT  ISRNumber=32  NumEventsToServe=1  EventsList={'on','EOC event','1';'off','Overflow event','2';'off','Custom event','3'}  SelectedEvents={'event1'}  TaskPriority=50  DisablePreemption=on  ClearInterruptFlagsAtEndOfEvent=on  InterruptDefinitionFile=$(TARGET_ROOT)/registry/interrupts/F2837xS_interrupts.xml  HardwareBoard=F2837x  EnableSimPort=off
      settings: LibrarySourceBlock=c2000lib/Scheduling/Hardware Interrupt
  Mux : Mux  Inputs=2
  HW_INT : Outport
  wires:
  HWI_ADCB1_INT/1 -> Mux/1
  HWI_SCIA_RX_INT/1 -> Mux/2
  Mux/1 -> HW_INT/1

== system mcb_pmsm_foc_I2C_f28379d/HW Interrupt/Simulation ==
  ADCINT1 : simulink/Ports & Subsystems/Function-Call Generator  sample_time=Ts  numberOfIterations=1  DisallowWideOutput=off
  Mux : Mux  Inputs=2
  SCI_Rx_INT : simulink/Ports & Subsystems/Function-Call Generator  sample_time=0.1  numberOfIterations=1  DisallowWideOutput=off
  HW_INT : Outport
  wires:
  SCI_Rx_INT/1 -> Mux/2
  ADCINT1/1 -> Mux/1
  Mux/1 -> HW_INT/1

== system mcb_pmsm_foc_I2C_f28379d/Hardware Init/Variant Subsystem ==
  In1 : Inport
  Code Generation : Subsystem  VariantControl=(codegen)
  Simulation : Subsystem  VariantControl=(sim)

== system mcb_pmsm_foc_I2C_f28379d/Heartbeat LED/Heartbeat LED ==
  In1 : Inport
  Code generation : Subsystem  VariantControl=(codegen)
  Simulation : Subsystem  VariantControl=(sim)

== system mcb_pmsm_foc_I2C_f28379d/Inverter and Motor - Plant Model/Codegeneration ==
  Duty_Cycles : Inport
  Ground : Ground
  Ground1 : Ground
  Terminator : Terminator
  Iab_fb_Sim : Outport  VectorParamsAs1DForOutWhenUnconnected=off
  Pos_fb_Sim : Outport  Port=2  VectorParamsAs1DForOutWhenUnconnected=off
  wires:
  Duty_Cycles/1 -> Terminator/1
  Ground/1 -> Iab_fb_Sim/1
  Ground1/1 -> Pos_fb_Sim/1

== system mcb_pmsm_foc_I2C_f28379d/Inverter and Motor - Plant Model/Simulation ==
  note: Note : Uncomment above subsystem to see vector plot
  Duty_Cycles : Inport
  Inverter : Subsystem
  Load_Profile (Torque) : Subsystem
  RT1 : RateTransition  Deterministic=off  OutPortSampleTime=Ts_simulink
  RT3 : RateTransition  Deterministic=off  OutPortSampleTime=Ts_simulink
  Rate Transition : RateTransition  Deterministic=off  OutPortSampleTime=Ts_motor
  Rate Transition1 : RateTransition  Deterministic=off  OutPortSampleTime=Ts_motor
  Sensor_Measurements : Subsystem
  Surface Mount PMSM : autolibpmsmexterior/Surface Mount PMSM  port_config=Torque  sim_type=Discrete  Ts=Ts_motor  P=pmsm.p  Rs=pmsm.Rs + inverter.R_board  Ldq_=pmsm.Ld  KConstText=Permanent flux linkage constant (lambda_pm):  lambda_pm=pmsm.FluxPM  Ke=159.9771  Kt=1.323  mechanical=[pmsm.J, pmsm.B, 0]  idq0=[0 0]  theta_init=0  omega_init=0  KConst=pmsm.FluxPM  lambda_pm_calc=pmsm.FluxPM  RefBlkName='autolibpmsmexterior/Surface Mount PMSM'  aMode=5  Ldq="[0.0002      0.0002]"
  Terminator : Terminator
  Vector Plot : Subsystem  Commented=on
  Iab_fb_Sim : Outport  VectorParamsAs1DForOutWhenUnconnected=off
  Pos_fb_Sim : Outport  Port=2  VectorParamsAs1DForOutWhenUnconnected=off
  wires:
  Load_Profile (Torque)/1(Load_Trq) -> Rate Transition1/1
  Rate Transition1/1 -> Surface Mount PMSM/1
  Surface Mount PMSM/2 -> RT1/1  "Iabc"
  Duty_Cycles/1 -> Inverter/1(Duty_abc)
  Surface Mount PMSM/3 -> Terminator/1
  Inverter/1(Vabc) -> Rate Transition/1
  Rate Transition/1 -> Vector Plot/2(Vabc), Surface Mount PMSM/2
  Surface Mount PMSM/1 -> RT3/1
  RT1/1 -> Vector Plot/1(Iabc), Sensor_Measurements/2(PhaseCurr)
  ? -> Vector Plot/3(Theta_mech)
  RT3/1 -> Sensor_Measurements/1(Info)
  Sensor_Measurements/1(Iab meas ADC) -> Iab_fb_Sim/1
  Sensor_Measurements/2(Pos_mech) -> Pos_fb_Sim/1

== system mcb_pmsm_foc_I2C_f28379d/Serial Receive/Data_Conditioning_Rx ==
  In1 : Inport
  Data_Type_Fixed_Point : Subsystem  VariantControl=~isequal(dataType, 'single')
  Data_Type_Float : Subsystem  VariantControl=isequal(dataType, 'single')
  Desired Speed : Outport
  Out2 : Outport  Port=2

== system mcb_pmsm_foc_I2C_f28379d/Serial Receive/SCI_Rx ==
  Code Generation : Subsystem  Variant=on  VariantControl=(codegen)
  Simulation : Subsystem  VariantControl=(sim)
  Data : Outport

== system mcb_pmsm_foc_I2C_f28379d/Serial Receive/unParse ==
  Data : Inport
  Bitwise Operator : simulink/Logic and Bit Operations/Bitwise Operator  logicop=AND  UseBitMask=on  BitMask=hex2dec('0001')  BitMaskRealWorld=Stored Integer
  Bitwise Operator1 : simulink/Logic and Bit Operations/Bitwise Operator  logicop=AND  UseBitMask=on  BitMask=hex2dec('00F0')  BitMaskRealWorld=Stored Integer
  Bitwise Operator2 : simulink/Logic and Bit Operations/Bitwise Operator  logicop=AND  UseBitMask=on  BitMask=hex2dec('0002')  BitMaskRealWorld=Stored Integer
  Data Type Conversion1 : DataTypeConversion  OutDataTypeStr=uint16  RndMeth=Simplest  SaturateOnIntegerOverflow=off
  Data Type Conversion3 : DataTypeConversion  OutDataTypeStr=boolean  RndMeth=Simplest  SaturateOnIntegerOverflow=off
  Data Type Conversion4 : DataTypeConversion  OutDataTypeStr=uint16  RndMeth=Simplest  SaturateOnIntegerOverflow=off
  Shift Arithmetic1 : ArithShift  BitShiftNumber=4
  Shift Arithmetic2 : ArithShift  BitShiftNumber=1
  Enable_PWM : Outport
  Debug_signals : Outport  Port=2
  Control_Mode : Outport  Port=3
  wires:
  Bitwise Operator1/1 -> Shift Arithmetic1/1
  Data/1 -> Bitwise Operator2/1, Bitwise Operator/1, Bitwise Operator1/1
  Bitwise Operator/1 -> Data Type Conversion3/1
  Data Type Conversion4/1 -> Debug_signals/1
  Shift Arithmetic1/1 -> Data Type Conversion4/1
  Data Type Conversion3/1 -> Enable_PWM/1
  Data Type Conversion1/1 -> Control_Mode/1
  Shift Arithmetic2/1 -> Data Type Conversion1/1
  Bitwise Operator2/1 -> Shift Arithmetic2/1

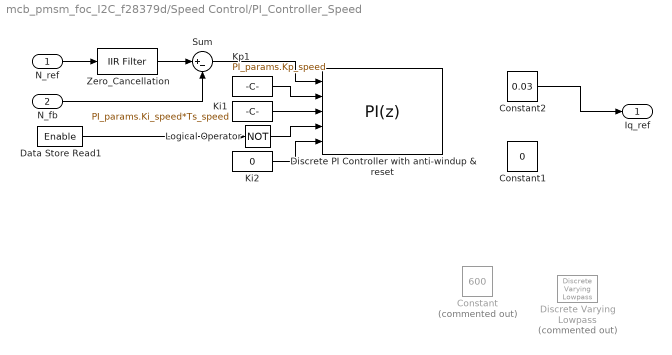
== system mcb_pmsm_foc_I2C_f28379d/Speed Control/PI_Controller_Speed ==
  N_ref : Inport
  N_fb : Inport  Port=2
  Constant : Constant  Commented=on  Value=600
  Constant1 : Constant  Value=0  OutDataTypeStr=single
  Constant2 : Constant  Value=0.03  OutDataTypeStr=single
  Data Store Read1 : DataStoreRead  DataStoreName=Enable  IndexOptions=Index vector (dialog)  Indices=1  OutputSizes=1
  Discrete PI Controller with anti-windup & reset : slpidlib/PID Controller  Controller=PI  Form=Parallel  TimeDomain=Discrete-time  UseExternalTs=off  SampleTime=-1  IntegratorMethod=Forward Euler  FilterMethod=Forward Euler  ControllerParametersSource=external  P=1  I=1  UseKiTs=on  D=0  N=100  UseFilter=on  TunerSelectOption=Transfer Function Based (PID Tuner App)  InitialConditionSource=external  InitialConditionForIntegrator=0  InitialConditionForFilter=0  DifferentiatorICPrevScaledInput=0  ExternalReset=level  TrackingMode=off  Kt=1  LimitOutput=on  SatLimitsSource=internal  UpperSaturationLimit=1  LowerSaturationLimit=-1  LinearizeAsGain=on  AntiWindupMode=clamping  Kb=1  LimitIntegrator=off  UpperIntegratorSaturationLimit=inf  LowerIntegratorSaturationLimit=-inf  RndMeth=Simplest  POutMin=[]  POutMax=[]  IOutMin=[]  IOutMax=[]  DOutMin=[]  DOutMax=[]  NOutMin=[]  NOutMax=[]  SumOutMin=[]  SumOutMax=[]  SaturationOutDataTypeStr=Inherit: Inherit via back propagation  SaturationOutMin=[]  SaturationOutMax=[]  PParamMin=[]  PParamMax=[]  IParamMin=[]  IParamMax=[]  DParamMin=[]  DParamMax=[]  NParamMin=[]  NParamMax=[]  KbParamMin=[]  KbParamMax=[]  KtParamMin=[]  KtParamMax=[]  KbOutMin=[]  KbOutMax=[]  KtOutMin=[]  KtOutMax=[]  IntegratorOutMin=[]  IntegratorOutMax=[]  FilterOutMin=[]  FilterOutMax=[]  SumI1OutMin=[]  SumI1OutMax=[]  SumI2OutMin=[]  SumI2OutMax=[]  SumI3OutMin=[]  SumI3OutMax=[]  SumI4OutMin=[]  SumI4OutMax=[]  SumDOutMin=[]  SumDOutMax=[]  DifferentiatorOutMin=[]  DifferentiatorOutMax=[]  FilterDiffOutCoefMin=[]  FilterDiffOutCoefMax=[]  ReciprocalOutMin=[]  ReciprocalOutMax=[]  SumDenOutMin=[]  SumDenOutMax=[]  SumNumOutMin=[]  SumNumOutMax=[]  DivideOutMin=[]  DivideOutMax=[]  UdiffTsProdOutMin=[]  UdiffTsProdOutMax=[]  NTsProdOutMin=[]  NTsProdOutMax=[]  UintegralTsProdOutMin=[]  UintegralTsProdOutMax=[]  UngainTsProdOutMin=[]  UngainTsProdOutMax=[]  ClampingZeroOutDataTypeStr=Inherit: Inherit via back propagation  ClampingZeroOutMin=[]  ClampingZeroOutMax=[]  FilterDenConstantOutDataTypeStr=Inherit: Inherit via back propagation  FilterDenConstantOutMin=[]  FilterDenConstantOutMax=[]  PCopyOutDataTypeStr=Inherit: Inherit via back propagation  PCopyOutMin=[]  PCopyOutMax=[]  NCopyOutDataTypeStr=Inherit: Inherit via back propagation  NCopyOutMin=[]  NCopyOutMax=[]  IntegratorContinuousStateAttributes=''  IntegratorStateMustResolveToSignalObject=off  IntegratorRTWStateStorageClass=Auto  FilterContinuousStateAttributes=''  FilterStateMustResolveToSignalObject=off  FilterRTWStateStorageClass=Auto  ParallelPVariant=ExternalParameters  IdealPVariant=Disabled  IVariant=ExternalParameters  DVariant=Disabled  IntegratorVariant=Discrete  SatVariant=Enabled  AWVariant=DiscClampingParallel  PCopyVariant=Disabled  TRVariant=Disabled  FdbkBlocksVariant=Forward  IdealPFdbkVariant=Disabled  SatFdbkVariant=Disabled  DerivativeFilterVariant=Disabled  NVariant=Disabled  NCopyVariant=Disabled_SignalSpec  FilterICVariant=Disabled  IntegratorICVariant=ExternalICs  ExternalResetVariant=ExternalReset  TRSumVariant=Passthrough  SumFdbkVariant=Disabled  SumVariant=Sum_PI  TsampFilterVariant=InternalTs  TsampNgainVariant=Passthrough  TsampIntegralVariant=Disabled_SignalSpec  ExternalSaturationOutDataTypeStr=Inherit: Same as second input
      settings: LibrarySourceBlock=mcbcontrolslib/PI Controller
  Discrete Varying Lowpass : cstblocks/Linear Parameter Varying/Discrete Varying Lowpass  Commented=on  N=1  w0=0  Ts=1e-3
  Ki1 : Constant  Value=PI_params.Ki_speed*Ts_speed  OutDataTypeStr=dataType  SampleTime=-1
  Ki2 : Constant  Value=0  OutDataTypeStr=dataType  SampleTime=-1
  Kp1 : Constant  Value=PI_params.Kp_speed  OutDataTypeStr=dataType  SampleTime=-1
  Logical Operator : Logic  Operator=NOT  IconShape=distinctive  AllPortsSameDT=off  OutDataTypeStr=boolean
  Sum : Sum  Inputs=|+-  OutDataTypeStr=Inherit: Same as first input
  Zero_Cancellation : mcbcontrolslib/IIR Filter  VariantControl=Low Pass Filter  VariantSelect=Low-pass  Filter_constant=0.01*(Ts_speed/Ts)  advancedSettings=off  Ts=50e-6  cutOff_freq=353.6777
  Iq_ref : Outport  VectorParamsAs1DForOutWhenUnconnected=off
  wires:
  Ki1/1 -> Discrete PI Controller with anti-windup & reset/3
  Kp1/1 -> Discrete PI Controller with anti-windup & reset/2
  N_fb/1 -> Sum/2
  N_ref/1 -> Zero_Cancellation/1
  Sum/1 -> Discrete PI Controller with anti-windup & reset/1
  Logical Operator/1 -> Discrete PI Controller with anti-windup & reset/4
  Ki2/1 -> Discrete PI Controller with anti-windup & reset/5
  Data Store Read1/1 -> Logical Operator/1
  Zero_Cancellation/1 -> Sum/1
  ? -> Discrete Varying Lowpass/1  "Iq_fb"
  Constant2/1 -> Iq_ref/1
